simulink model "AGV_simulate"  (R2025b)
settings: Solver=VariableStepAuto  StartTime=0.0  StopTime=20  RelTol=1e-3
libraries: simulink x1
settings Model: Creator=余陶健喆  LastModifiedBy=31586
settings DebuggingCC: AlgebraicLoopMsg=error

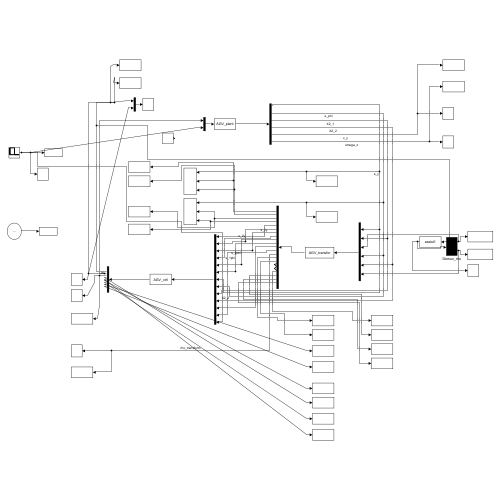
[thumbnail: Simulink's stored preview of the top-level diagram]
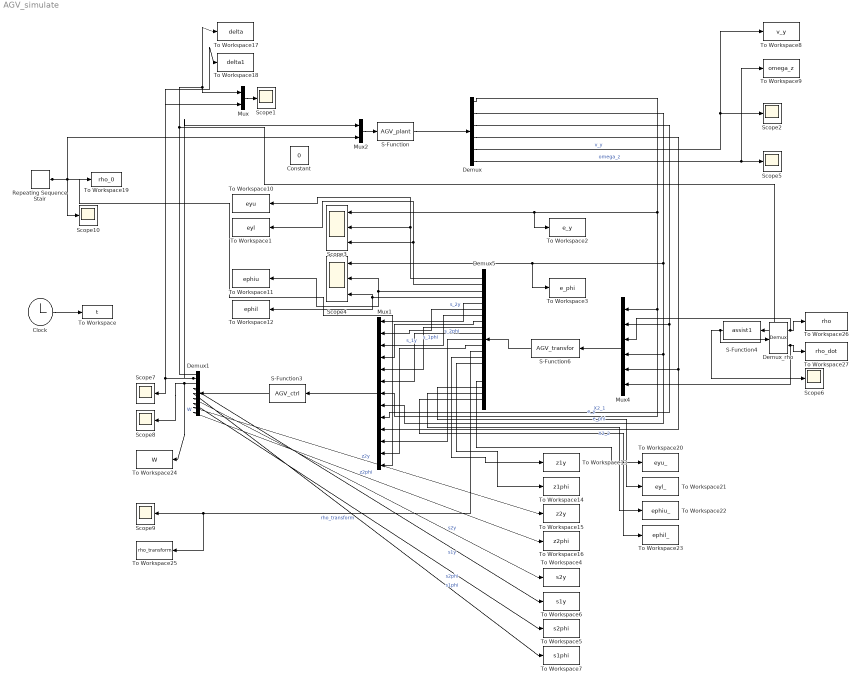
== system AGV_simulate ==
  Clock : Clock
      settings: Decimation=40
  Constant : Constant  Value=0
  Demux : Demux  Outputs=6
  Demux1 : Demux  Outputs=9
  Demux5 : Demux  Outputs=21
  Demux_rho : Demux  Outputs=2
  Mux : Mux  Inputs=2
  Mux1 : Mux  Inputs=13
  Mux2 : Mux  Inputs=2
  Mux4 : Mux  Inputs=6
  Repeating Sequence Stair : simulink/Sources/Repeating Sequence Stair  OutValues=[0 0 0.002 0.002 0.002 0.002 0.002 0.002 0.002 0.002 0 0 0 0 0 0 0 0 0 0]  tsamp=1  OutMin=[]  OutMax=[]  OutDataTypeStr=double  OutputDataTypeScalingMode=double  OutDataType=fixdt(0,8)  ConRadixGroup=Best Precision: Vector-wise  OutScaling=2^-12
  S-Function : S-Function  FunctionName=AGV_plant  SFunctionDeploymentMode=off  EnableBusSupport=off
  S-Function3 : S-Function  FunctionName=AGV_ctrl  SFunctionDeploymentMode=off  EnableBusSupport=off
  S-Function4 : S-Function  FunctionName=assist1  SFunctionDeploymentMode=off  EnableBusSupport=off
  S-Function6 : S-Function  FunctionName=AGV_transfor  SFunctionDeploymentMode=off  EnableBusSupport=off
  Scope{1..2,5..10} (8 alike) : Scope
      Scope1 settings: ActiveDisplayYMinimum=-4.0692536530838117  ActiveDisplayYMaximum=3.0278687460146125
      Scope10 settings: ActiveDisplayYMinimum=-0.027394798352207671  ActiveDisplayYMaximum=0.022114058231530266  DataLoggingVariableName=ScopeData9
      Scope2 settings: ActiveDisplayYMinimum=-0.6302271852844904  ActiveDisplayYMaximum=0.56114738295653732
      Scope5 settings: ActiveDisplayYMinimum=-0.38999049248441087  ActiveDisplayYMaximum=0.41040952711934142  DataLoggingVariableName=ScopeData2
      Scope6 settings: ActiveDisplayYMinimum=-18.326211488105606  ActiveDisplayYMaximum=28.74441705952875  DataLoggingVariableName=ScopeData5
      Scope7 settings: ActiveDisplayYMinimum=-0.00084853983296151458  ActiveDisplayYMaximum=0.28942053056735983  DataLoggingVariableName=ScopeData6
      Scope8 settings: ActiveDisplayYMinimum=-1.8640662428629926  ActiveDisplayYMaximum=4.82103164327777  DataLoggingVariableName=ScopeData7
      Scope9 settings: ActiveDisplayYMinimum=-1.2592769233717198  ActiveDisplayYMaximum=4.0863310000077258  DataLoggingVariableName=ScopeData8
  Scope3 : Scope  NumInputPorts=3
      settings: ActiveDisplayYMinimum=-0.49603566640977825  ActiveDisplayYMaximum=0.436154486159952  DataLoggingVariableName=ScopeData3
  Scope4 : Scope  NumInputPorts=3
      settings: ActiveDisplayYMinimum=-0.30680106774737592  ActiveDisplayYMaximum=0.24540821488641756  DataLoggingVariableName=ScopeData4
  To Workspace : ToWorkspace  VariableName=t  SampleTime=-1
  To Workspace1 : ToWorkspace  VariableName=eyl  SampleTime=-1
  To Workspace10 : ToWorkspace  VariableName=eyu  SampleTime=-1
  To Workspace11 : ToWorkspace  VariableName=ephiu  SampleTime=-1
  To Workspace12 : ToWorkspace  VariableName=ephil  SampleTime=-1
  To Workspace13 : ToWorkspace  VariableName=z1y  SampleTime=-1
  To Workspace14 : ToWorkspace  VariableName=z1phi  SampleTime=-1
  To Workspace15 : ToWorkspace  VariableName=z2y  SampleTime=-1
  To Workspace16 : ToWorkspace  VariableName=z2phi  SampleTime=-1
  To Workspace17 : ToWorkspace  VariableName=delta  SampleTime=-1
  To Workspace18 : ToWorkspace  VariableName=delta1  SampleTime=-1
  To Workspace19 : ToWorkspace  VariableName=rho_0  SaveFormat=Timeseries  SampleTime=-1
  To Workspace2 : ToWorkspace  VariableName=e_y  SampleTime=-1
  To Workspace20 : ToWorkspace  VariableName=eyu_  SampleTime=-1
  To Workspace21 : ToWorkspace  VariableName=eyl_  SampleTime=-1
  To Workspace22 : ToWorkspace  VariableName=ephiu_  SampleTime=-1
  To Workspace23 : ToWorkspace  VariableName=ephil_  SampleTime=-1
  To Workspace24 : ToWorkspace  VariableName=W  SampleTime=-1
  To Workspace25 : ToWorkspace  VariableName=rho_transform  SampleTime=-1
  To Workspace26 : ToWorkspace  VariableName=rho  SampleTime=-1
  To Workspace27 : ToWorkspace  VariableName=rho_dot  SampleTime=-1
  To Workspace3 : ToWorkspace  VariableName=e_phi  SampleTime=-1
  To Workspace4 : ToWorkspace  VariableName=s2y  SampleTime=-1
  To Workspace5 : ToWorkspace  VariableName=s2phi  SampleTime=-1
  To Workspace6 : ToWorkspace  VariableName=s1y  SampleTime=-1
  To Workspace7 : ToWorkspace  VariableName=s1phi  SampleTime=-1
  To Workspace8 : ToWorkspace  VariableName=v_y  SampleTime=-1
  To Workspace9 : ToWorkspace  VariableName=omega_z  SampleTime=-1
  wires:
  S-Function/1 -> Demux/1
  Demux/1 -> Mux1/7, Mux4/1, To Workspace2/1, Scope3/1  "e_y"
  Demux/2 -> Mux1/8, Mux4/4, To Workspace3/1, Scope4/1  "e_phi"
  Demux/3 -> Mux1/9, Mux4/2  "X2_1"
  Demux/4 -> Mux1/10, Mux4/5  "X2_2"
  Mux1/1 -> S-Function3/1
  Mux4/1 -> S-Function6/1
  S-Function6/1 -> Demux5/1
  Demux5/7 -> Mux1/3  "s_1y"
  Demux5/10 -> Mux1/6  "s_1phi"
  Demux5/5 -> Mux1/1
  Demux5/8 -> Mux1/4
  Demux5/1 -> To Workspace10/1, Scope3/2
  Demux5/2 -> To Workspace1/1, Scope3/3
  Demux5/3 -> Scope4/2, To Workspace11/1
  Demux5/4 -> To Workspace12/1, Scope4/3
  Demux5/6 -> Mux1/2  "s_2y"
  Demux5/9 -> Mux1/5  "s_2phi"
  S-Function4/1 -> Scope6/1, Demux_rho/1
  Demux5/13 -> To Workspace25/1, Scope9/1  "rho_transform"
  Demux5/11 -> Mux1/11
  Demux5/12 -> Mux1/12
  Demux/5 -> Scope2/1, To Workspace8/1  "v_y"
  Demux/6 -> To Workspace9/1, Scope5/1  "omega_z"
  S-Function3/1 -> Demux1/1
  Demux1/1 -> To Workspace17/1, Mux/1, S-Function4/1
  Demux1/2 -> To Workspace18/1, Scope7/1, Mux/2, Mux2/1
  Demux1/3 -> To Workspace24/1, Scope8/1  "W"
  Mux/1 -> Scope1/1
  Demux1/4 -> To Workspace6/1  "s1y"
  Demux1/5 -> To Workspace7/1  "s1phi"
  Demux1/6 -> To Workspace4/1  "s2y"
  Demux1/7 -> To Workspace5/1  "s2phi"
  Demux1/8 -> To Workspace15/1  "z2y"
  Demux1/9 -> To Workspace16/1  "z2phi"
  Mux2/1 -> S-Function/1
  Repeating Sequence Stair/1 -> To Workspace19/1, Scope10/1, Mux2/2, Mux1/13
  Clock/1 -> To Workspace/1
  Demux5/14 -> To Workspace13/1
  Demux5/15 -> To Workspace14/1
  Demux5/18 -> To Workspace20/1
  Demux5/19 -> To Workspace21/1
  Demux5/20 -> To Workspace22/1
  Demux5/21 -> To Workspace23/1
  Demux_rho/1 -> Mux4/3, To Workspace26/1
  Demux_rho/2 -> Mux4/6, To Workspace27/1
